simulink model "EnduranceSim"  (R2026a)
settings: Solver=VariableStepAuto  StopTime=1e6  MaxStep=10
undefined symbols (not defined in the file or in its folder): capacity_Ah, V_nom
libraries: simulink x1
settings Model: Creator=potlo  LastModifiedBy=potlo

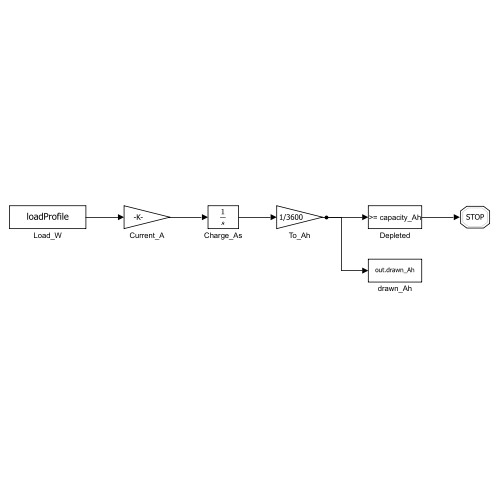
[thumbnail: Simulink's stored preview of the top-level diagram]
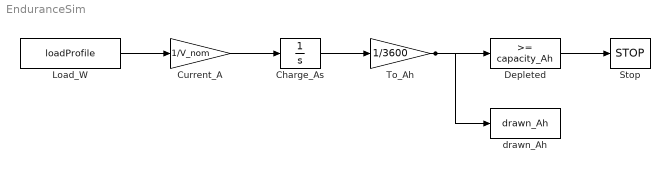
== system EnduranceSim ==
  Charge_As : Integrator
  Current_A : Gain  Gain=1/V_nom
  Depleted : simulink/Logic and Bit Operations/Compare To Constant  relop=>=  const=capacity_Ah  OutDataTypeStr=boolean
  Load_W : FromWorkspace  VariableName=loadProfile  OutputAfterFinalValue=Holding final value
  Stop : Stop
  To_Ah : Gain  Gain=1/3600
  drawn_Ah : ToWorkspace  VariableName=drawn_Ah  SaveFormat=Timeseries  SampleTime=-1
  wires:
  Load_W/1 -> Current_A/1
  Current_A/1 -> Charge_As/1
  Charge_As/1 -> To_Ah/1
  To_Ah/1 -> Depleted/1, drawn_Ah/1
  Depleted/1 -> Stop/1
